simulink model "simulink7"  (R2025b)
settings: Solver=ode45  StartTime=0.0  StopTime=10  MaxStep=2^-5  RelTol=1e-3
settings Model: Creator=mizula  LastModifiedBy=mizula

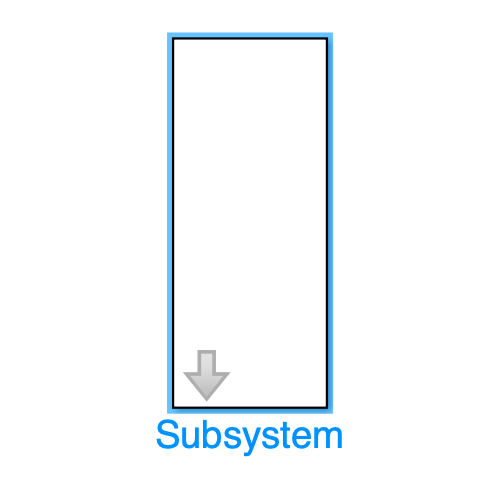
[thumbnail: Simulink's stored preview of the top-level diagram]
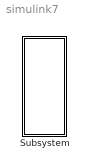
== system simulink7 ==
  Subsystem : Subsystem  mask{g=9.81, k1=2, k2=1, m1=1, m2=2, l1=1, l2=2, th1=80, th2=150, th3=0, th4=0}

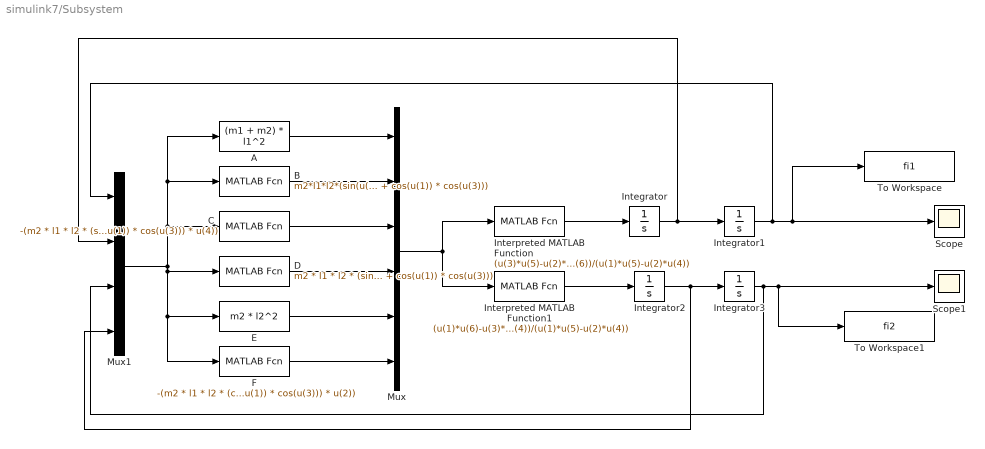
== system simulink7/Subsystem ==
  A : MATLABFcn  MATLABFcn=(m1 + m2) * l1^2
  B : MATLABFcn  MATLABFcn=m2*l1*l2*(sin(u(1)) * sin(u(3)) + cos(u(1)) * cos(u(3)))
  C : MATLABFcn  MATLABFcn=-(m2 * l1 * l2 * (sin(u(1)) * cos(u(3)) - cos(u(1)) * sin(u(3))) * u(4)^2 + (m1 + m2) * g * l1 * sin(u(1)) + k1 * l1^2 * u(2) + k2 * l1 * l2 * (sin(u(1)) * sin(u(3)) + cos(u(1)) * cos(u(3))) * u(4))
  D : MATLABFcn  MATLABFcn=m2 * l1 * l2 * (sin(u(1)) * sin(u(3)) + cos(u(1)) * cos(u(3)))
  E : MATLABFcn  MATLABFcn=m2 * l2^2
  F : MATLABFcn  MATLABFcn=-(m2 * l1 * l2 * (cos(u(1)) * sin(u(3)) - sin(u(1)) * cos(u(3))) * u(2)^2 + m2 * g * l2 * sin(u(3)) + k2 * l2^2 * u(4) + k2 * l1 * l2 *(sin(u(1)) * sin(u(3)) + cos(u(1)) * cos(u(3))) * u(2))
  Integrator : Integrator  InitialCondition=th3*pi/180
  Integrator1 : Integrator  InitialCondition=th1*pi/180
  Integrator2 : Integrator  InitialCondition=th4*pi/180
  Integrator3 : Integrator  InitialCondition=th2*pi/180
  Interpreted MATLAB Function : MATLABFcn  MATLABFcn=(u(3)*u(5)-u(2)*u(6))/(u(1)*u(5)-u(2)*u(4))
  Interpreted MATLAB Function1 : MATLABFcn  MATLABFcn=(u(1)*u(6)-u(3)*u(4))/(u(1)*u(5)-u(2)*u(4))
  Mux : Mux  Inputs=6
  Mux1 : Mux
  Scope : Scope
      settings: ActiveDisplayYMinimum=-1  ActiveDisplayYMaximum=1
  Scope1 : Scope
      settings: ActiveDisplayYMinimum=-1  ActiveDisplayYMaximum=1
  To Workspace : ToWorkspace  VariableName=fi1  SaveFormat=Timeseries  SampleTime=-1
  To Workspace1 : ToWorkspace  VariableName=fi2  SaveFormat=Timeseries  SampleTime=-1
  wires:
  D/1 -> Mux/4
  C/1 -> Mux/3
  B/1 -> Mux/2
  F/1 -> Mux/6
  Integrator/1 -> Mux1/2, Integrator1/1
  A/1 -> Mux/1
  Integrator3/1 -> Mux1/3, To Workspace1/1, Scope1/1
  Mux/1 -> Interpreted MATLAB Function1/1, Interpreted MATLAB Function/1
  Integrator2/1 -> Mux1/4, Integrator3/1
  Interpreted MATLAB Function/1 -> Integrator/1
  Mux1/1 -> F/1, E/1, D/1, C/1, A/1, B/1
  Integrator1/1 -> Mux1/1, Scope/1, To Workspace/1
  Interpreted MATLAB Function1/1 -> Integrator2/1
  E/1 -> Mux/5
